simulink model "ssp3"  (R2014a)
settings: Solver=VariableStepDiscrete  StartTime=0.0  StopTime=10.0  RelTol=1e-3
libraries: dspvision x2
settings Model: Creator=root  LastModifiedBy=root

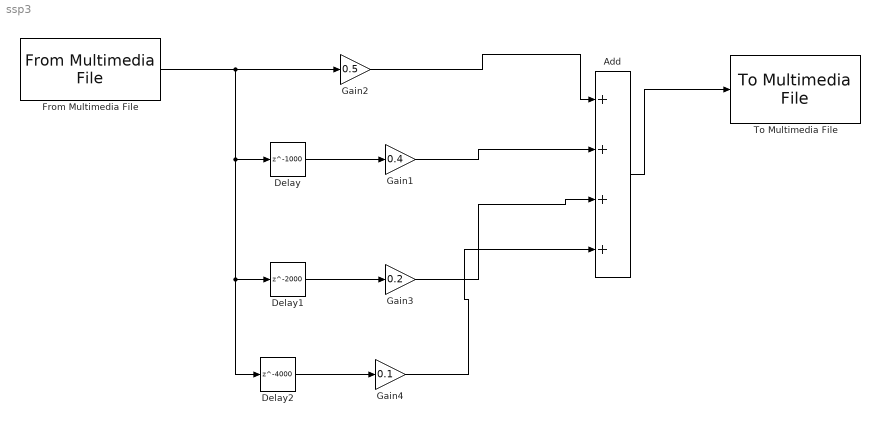
== system ssp3 ==
  Add : Sum  Inputs=++++
  Delay : Delay  DelayLength=1000  InitialCondition=0
  Delay1 : Delay  DelayLength=2000  InitialCondition=0
  Delay2 : Delay  DelayLength=4000  InitialCondition=0
  From Multimedia File : dspvision/From Multimedia File  inputFilename=/home/brjathu/hawking01.wav  loop=on  numPlays=inf  outputStreams=Audio only  videoDataType=int16  audioDataType=int16  inheritSampleTime=on  userDefinedSampleTime=1/30  noAudioOutput=off  isIntensityVideo=off  fourcc=RGB  colorVideoFormat=One multidimensional signal  outputEOF=off  dataOrg=Column-major  audioFrameSize=1  computeAudioFrameSize=off  outSamplingMode=Sample based
  Gain1 : Gain  Gain=0.4  OutDataTypeStr=int16
  Gain2 : Gain  Gain=0.5  OutDataTypeStr=int16
  Gain3 : Gain  Gain=0.2  OutDataTypeStr=int16
  Gain4 : Gain  Gain=0.1  OutDataTypeStr=int16
  To Multimedia File : dspvision/To Multimedia File  outputFilename=output1.wav  streamSelection=Audio only  videoCompressor=None (uncompressed)  audioCompressor=None (uncompressed)  imagePorts=One multidimensional signal  fileType=WAV  audioDatatype=Determine from input data type  fourcc=RGB  videoQuality=75  mj2000CompFactor=10
  wires:
  Delay/1 -> Gain1/1
  Gain2/1 -> Add/1
  Gain1/1 -> Add/2
  Add/1 -> To Multimedia File/1
  From Multimedia File/1 -> Gain2/1, Delay2/1, Delay1/1, Delay/1
  Delay1/1 -> Gain3/1
  Gain3/1 -> Add/3
  Delay2/1 -> Gain4/1
  Gain4/1 -> Add/4
